simulink model "JoystickDemo"  (R2024b)
settings: Solver=VariableStepAuto  StartTime=0.0  StopTime=t_final  RelTol=1e-3
values from neighbouring files (symbols this model uses):
  dt = 1/50    (= 0.02)    [Initializemodel.m]
libraries: aerolibanimutils x2
settings Model: Creator=satvik_sh  LastModifiedBy=satvik_sh

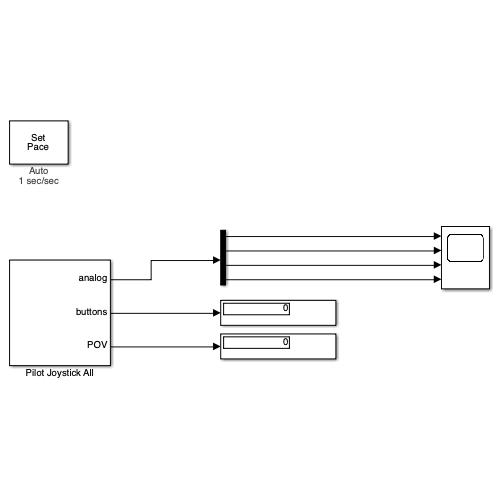
[thumbnail: Simulink's stored preview of the top-level diagram]
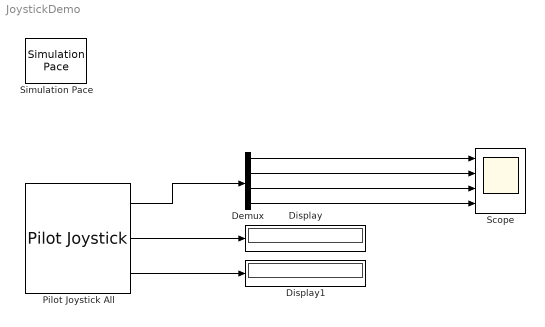
== system JoystickDemo ==
  Demux : Demux
  Display : Display
  Display1 : Display
  Pilot Joystick All : aerolibanimutils/Pilot Joystick  JoystickID=Joystick1  OutputConfiguration=AllOutputs  SampleTime=dt
      settings: LibrarySourceBlock=aerolibanimutils/Pilot Joystick All
  Scope : Scope  NumInputPorts=4
  Simulation Pace : aerolibanimutils/Simulation Pace  SimulationPace=1  SleepMode=Auto  OutputPaceError=off  SampleTime=dt
  wires:
  Pilot Joystick All/2 -> Display/1
  Pilot Joystick All/3 -> Display1/1
  Pilot Joystick All/1 -> Demux/1
  Demux/1 -> Scope/1
  Demux/2 -> Scope/2
  Demux/3 -> Scope/3
  Demux/4 -> Scope/4
